simulink model "IEEE123_4subsystem"  (R2022b)
settings: Solver=ode4  StartTime=0.0  StopTime=inf  FixedStep=Ts  MaxStep=1e-4  RelTol=1e-3
PreLoadFcn:
  | Ts = 50e-6;
PostLoadFcn:
  | Ts = 50e-6;
InitFcn:
  | %%%%%%%%%%%%%%%%%%%%%%%%
  | % Simulation data for the IEEE 123 Node Test Feeder model
  | %%%%%%%%%%%%%%%%%%%%%%%
  | 
  | % miles/km
  | mi2km = 1.60934;
  | 
  | % feet to km
  | ft2km = 0.0003048;
  | 
  | % microsiemens to Farads
  | ms2F = 1/2/pi/60*1e-6;
  | 
  | %% Configuration 1 - series reactance - ohm/mile
  | 
  | R_1 = [0.4576 0.1560 0.1535;0.1560 0.4666 0.1580;0.1535 0.1580 0.4615];
  | X_1 = [1.0780 0.5017 0.3849;0.5017 1.0482 0.4236;0.3849 0.4236 1.0651];
  | 
  | % charging susceptance - microsiemens/mile
  | 
  | B_1 = [5.6765 -1.8319 -0.6982;-1.8319 5.9809 -1.1645;-0.6982 -1.1645 5.3971];
  | 
  | % convert for SPS
  | 
  | R_1 = R_1/mi2km;
  | 
  | Rs_1=(R_1(1,1)+R_1(2,2)+R_1(3,3))/3;
  | Rm_1=(R_1(1,2)+R_1(1,3)+R_1(2,3))/3;
  | R1_1=Rs_1-Rm_1;
  | R0_1=Rs_1+2*Rm_1;
  | 
  | L_1 = X_1/mi2km/2/pi/60;
  | 
  | Ls_1=(L_1(1,1)+L_1(2,2)+L_1(3,3))/3;
  | Lm_1=(L_1(1,2)+L_1(1,3)+L_1(2,3))/3;
  | L1_1=Ls_1-Lm_1;
  | L0_1=Ls_1+2*Lm_1;
  | 
  | C_1 = B_1/mi2km*ms2F;
  | 
  | Cs_1=(C_1(1,1)+C_1(2,2)+C_1(3,3))/3;
  | Cm_1=(C_1(1,2)+C_1(1,3)+C_1(2,3))/3;
  | C1_1=Cs_1-Cm_1;
  | C0_1=Cs_1+2*Cm_1;
  | 
  | 
  | %% Configuration 2 - series reactance - ohm/mile
  | 
  | R_2 = [0.4666 0.1580 0.1560;0.1580 0.4615 0.1535;0.1560 0.1535 0.4576];
  | X_2 = [1.0482 0.4236 0.5017;0.4236 1.0651 0.3849;0.5017 0.3849 1.0780];
  | 
  | % charging susceptance - microsiemens/mile
  | 
  | B_2 = [5.9809 -1.1645 -1.8319;-1.1645 5.3971 -0.6982;-1.8319 -0.6982 5.6765];
  | 
  | % convert for SPS
  | 
  | R_2 = R_2/mi2km;
  | 
  | Rs_2=(R_2(1,1)+R_2(2,2)+R_2(3,3))/3;
  | ... (+341 lines)
undefined symbols (not defined in the file): D1, Delta, find_system, I, Left, MOV_segment9, powergui, Right, type, V, X
libraries: spsGroundLib x242, spsThreePhaseVIMeasurementLib x134, spsSeriesRLCBranchLib x107, spsSeriesRLCLoadLib x83, spsPiSectionLineLib x61, spsThreePhasePISectionLineLib x60, spsVoltageMeasurementLib x52, spsDCVoltageSourceLib x36, ssn_lib x28, artemis x24, spsACCurrentSourceLib x18, spsOnDelayLib x18
(part 11 of 15)

== system IEEE123_4subsystem/SM_123p/Regulator 1 Three Phase Ganged SVR/Single Phase SVR_A/Voltage Regulator Control/Tap Changer Control ==
  "Up " : Inport
  "Down " : Inport  Port=2
  Constant : Constant  Value=-1
  Constant1 : Constant
  Determine tap position : Subsystem
  Edge Detector : Subsystem  DialogController=POWERSYS.PowerSysDialog  mask(Edge Detector){model=Rising, ic=0}
      mask prompts: model "Edge:"; ic "Input at t = -eps:"
      mask help:
      | This block compares its present input to its previous input.
      |
      | If the input  is a logic signal (TRUE (1) or FALSE (0), the output is a one-step boolean signal TRUE  when  the specified edge (Rising, Falling or Either)  is detected.
      |
      | This block can also be used to detect the slope polarity of a continuous signal. For example, if the specified edge is  "Rising", the output is TRUE as long as the slope of the input signal is positive.
      |
      | The input value at time preceding t=0 is specified by the parameter "Input at t=-eps"
      mask init:
      | if model~=3,
      | 	x1 = (model -1)*20;
      |     x2 = (model -1)*60;
      | 	X1=[5,20,20,35]+25; Y1=[20+x2,20+x2,80-x2,80-x2];
      | 	X2=[5,20,35]+25;    Y2=[40+x1,60-x1,40+x1];
      | 	X3=[];X4=[];Y3=[];Y4=[];
      | else
      | 	x1 = 20;
      | 	x2 = 60;
      | 	X1=[5,20,20,35]+8; Y1=[20,20,80,80];
      | 	X2=[5,20,35]+8;    Y2=[40,60,40];
      | 	X3=[5,20,20,35]+53; Y3=[20+x2,20+x2,80-x2,80-x2];
      | 	X4=[5,20,35]+53;    Y4=[40+x1,60-x1,40+x1];
      | end
      | power_initmask();
      mask Help: This block is part of a subset of blocks in the Extras library that does not have documentation associated with it, other than the block mask description.
      mask TypeOptions model: Rising | Falling | Either
      mask Display: plot(0,0,100,100, X1,Y1,X2,Y2,X3,Y3,X4,Y4);
  Logical Operator : Logic  Operator=OR  AllPortsSameDT=off
  Logical Operator1 : Logic  AllPortsSameDT=off
  Mechanical Delay : TransportDelay  DelayTime=MecDelay  InitialOutput=InitialPosition  BufferSize=5120
  Memory : Memory  InitialCondition=1  InheritSampleTime=on
  Relational Operator : RelationalOperator  Operator===  OutDataTypeStr=float('double')  InputSameDT=off
  Switch : Switch  Threshold=0.5  InputSameDT=off
  TapNo : Outport  VectorParamsAs1DForOutWhenUnconnected=off
  Ready : Outport  Port=2  VectorParamsAs1DForOutWhenUnconnected=off
  wires:
  Edge Detector/1(Out) -> Logical Operator1/2
  Logical Operator/1 -> Edge Detector/1(In)
  Memory/1 -> Ready/1, Logical Operator1/1
  Relational Operator/1 -> Memory/1
  Determine tap position/1(TapNo) -> Relational Operator/1, Mechanical Delay/1
  Switch/1 -> Determine tap position/1(NewTap)
  Constant1/1 -> Switch/3
  Constant/1 -> Switch/1
  "Down "/1 -> Switch/2, Logical Operator/2
  "Up "/1 -> Logical Operator/1
  Logical Operator1/1 -> Determine tap position/Trigger
  Mechanical Delay/1 -> Relational Operator/2, TapNo/1

== system IEEE123_4subsystem/SM_123p/Regulator 1 Three Phase Ganged SVR/Single Phase SVR_A/Voltage Regulator Control/Voltage regulator ==
  Vmes (pu) : Inport
  Ready : Inport  Port=2
  RegOn : Inport  Port=3
  Dead Zone : DeadZone  LowerValue=-DeadBand/2  UpperValue=+DeadBand/2
  Discrete Variable Time Delay : spsDiscreteVariableTimeDelayLib/Discrete Variable Time Delay  MaxDelay=3/60+Ts  InitialValue=1  Ts=Ts  DFT=on
      settings: LibrarySourceBlock=|
      | sps_lib/Control/Discrete Variable
      | Time Delay
  Logical Operator : Logic  AllPortsSameDT=off
  Logical Operator1 : Logic  AllPortsSameDT=off
  On Delay : spsOnDelayLib/On Delay  DelayType=On delay  delay=TimeDelay  ic=0  Ts=Ts
  On Delay1 : spsOnDelayLib/On Delay  DelayType=On delay  delay=TimeDelay  ic=0  Ts=Ts
  Relational Operator : RelationalOperator  Operator=>  InputSameDT=off
  Relational Operator1 : RelationalOperator  Operator=<  InputSameDT=off
  Sum : Sum  Inputs=|+-  SaturateOnIntegerOverflow=on
  Switch : Switch  Threshold=1.5  InputSameDT=off
  Vref : Constant  Value=Vref
  Vref1 : Constant  Value=0
  Vref2 : Constant  Value=0
  Vref3 : Constant  Value=0
  Vref4 : Constant  Value=3/60
  Up : Outport  VectorParamsAs1DForOutWhenUnconnected=off
  Down : Outport  Port=2  VectorParamsAs1DForOutWhenUnconnected=off
  wires:
  Vref4/1 -> Discrete Variable Time Delay/2
  Discrete Variable Time Delay/1 -> Logical Operator/2, Logical Operator1/1
  Vref3/1 -> Relational Operator1/2
  On Delay1/1 -> Down/1
  Logical Operator1/1 -> On Delay1/1
  Relational Operator1/1 -> Logical Operator1/2
  On Delay/1 -> Up/1
  Logical Operator/1 -> On Delay/1
  Ready/1 -> Discrete Variable Time Delay/1
  Relational Operator/1 -> Logical Operator/1
  Vref1/1 -> Relational Operator/2
  Dead Zone/1 -> Relational Operator/1, Relational Operator1/1
  Vmes (pu)/1 -> Sum/2
  Vref/1 -> Sum/1
  Sum/1 -> Switch/1
  Switch/1 -> Dead Zone/1
  RegOn/1 -> Switch/2
  Vref2/1 -> Switch/3

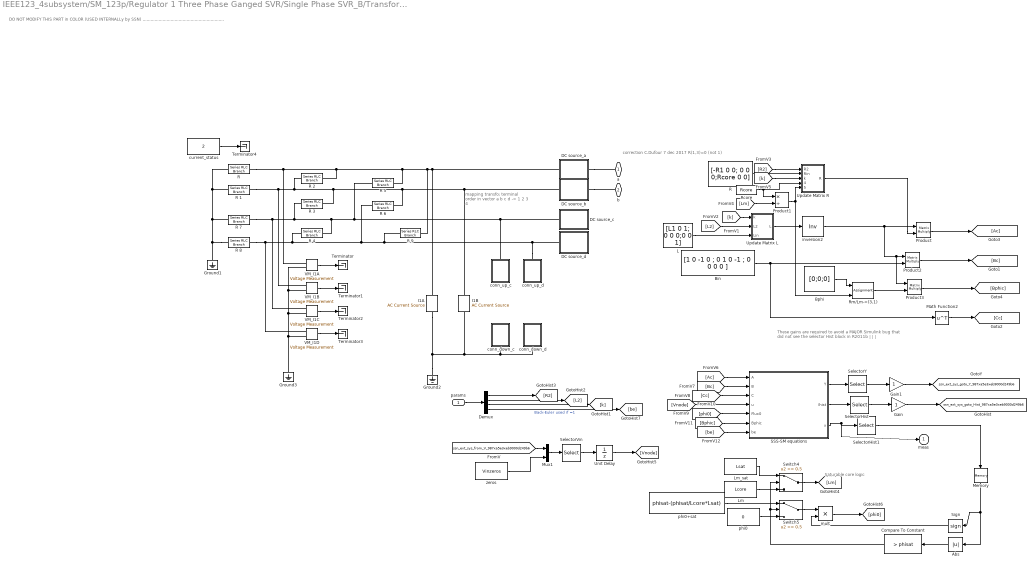
== system IEEE123_4subsystem/SM_123p/Regulator 1 Three Phase Ganged SVR/Single Phase SVR_B/Transformer with Taps/SSN OLTC xfo v2 ==
  note: correction C.Dufour 7 dec 2017 R(1,3)=0 (not 1)
  note: These gains are required to avoid a MAJOR Simulink bug
      | that did not see the selector Hist block in R2011b
      | |
      | |
      | |
  note: Saturable core logic
  note: DO NOT MODIFY THIS PART in COLOR (USED INTERNALLy by SSN) .............................................................
  note: mapping transfo:
      | terminal    order in vector
      | a b c d -> 1 2 3 4
  params : Inport
  Abs : Abs  SaturateOnIntegerOverflow=off
  Bin : Constant  Value="[1 0 -1  0 ; 0 1 0 -1 ; 0 0 0 0 ]"
  Bphi : Constant  Value=[0;0;0]  VectorParams1D=off
  Compare To Constant : simulink/Logic and Bit Operations/Compare To Constant  relop=>  const=phisat  OutDataTypeStr=uint8
  DC source_a : Subsystem  mask(SSN nodal point interface: DC-source){}
  DC source_b : Subsystem  mask(SSN nodal point interface: DC-source){}
  DC source_c : Subsystem  mask(SSN nodal point interface: DC-source){}
  DC source_d : Subsystem  mask(SSN nodal point interface: DC-source){}
  Demux : Demux
  Gain : Gain
  Gain1 : Gain
  Ground1 : spsGroundLib/Ground  LConnTagsString=a
  Ground2 : spsGroundLib/Ground  LConnTagsString=a
  Ground3 : spsGroundLib/Ground  LConnTagsString=a
  I1A : spsACCurrentSourceLib/AC Current Source  Amplitude=0  Phase=0  Frequency=1928.3746  SampleTime=0  Measurements=None
      settings: LibrarySourceBlock=sps_lib/Sources/AC Current Source
  I1B : spsACCurrentSourceLib/AC Current Source  Amplitude=0  Phase=0  Frequency=1928.3746  SampleTime=0  Measurements=None
      settings: LibrarySourceBlock=sps_lib/Sources/AC Current Source
  L : Constant  Value=[L1 0 1; 0 0 0;0 0 1]
  Lm : Constant  Value=Lcore
  Lm_sat : Constant  Value=Lsat
  Math Function2 : Math  Operator=transpose  SignedPower=on
  Memory : Memory
  Mux1 : Mux  Inputs=2
  Product : Product  Multiplication=Matrix(*)  RndMeth=Zero
  Product1 : Product  Inputs=*/  RndMeth=Zero
  Product2 : Product  Multiplication=Matrix(*)  RndMeth=Zero
  Product3 : Product  Multiplication=Matrix(*)  RndMeth=Zero
  R : Constant  Value=[-R1 0 0; 0 0 0;Rcore 0 0]
  R {,1..9} (10 alike) : spsSeriesRLCBranchLib/Series RLC Branch  LConnTagsString=__new0  RConnTagsString=__new0  BranchType=R  Resistance=1.23456789  Inductance=.5  SetiL0=off  InitialCurrent=0  Capacitance=1.0  Setx0=off  InitialVoltage=0  Measurements=None
  Rcore : Constant  Value=Rcore
  "Rm/Lm->(3,1) " : Assignment  NumberOfDimensions=2  IndexOptions=Index vector (dialog),Index vector (dialog)  Indices=3,1  OutputSizes=1,1
  SSS-SM equations : Subsystem
  SelectorHist : Selector  InputPortWidth=4  IndexOptions=Index vector (dialog)  Indices=hist_sel  OutputSizes=1
  SelectorHist1 : Selector  InputPortWidth=3  IndexOptions=Index vector (dialog)  Indices=3  OutputSizes=1
  SelectorVin : Selector  InputPortWidth=5  IndexOptions=Index vector (dialog)  Indices=vin_sel  OutputSizes=1
  SelectorY : Selector  NumberOfDimensions=2  InputPortWidth=4  IndexOptions=Index vector (dialog),Index vector (dialog)  Indices=hist_sel,hist_sel  OutputSizes=1,1
  Sign : Signum
  Switch4 : Switch  Threshold=0.5  SaturateOnIntegerOverflow=off  InputSameDT=off
  Switch5 : Switch  Threshold=0.5  SaturateOnIntegerOverflow=off  InputSameDT=off
  Terminator{,1..4} (5 alike) : Terminator
  Unit Delay : UnitDelay  SampleTime=Ts  HasFrameUpgradeWarning=on
  Update Matrix L : Subsystem
  Update Matrix R : Subsystem
  VM_I1A : spsVoltageMeasurementLib/Voltage Measurement  PhasorSimulation=off  OutputType=Complex  PSBequivalent=0
  VM_I1B : spsVoltageMeasurementLib/Voltage Measurement  PhasorSimulation=off  OutputType=Complex  PSBequivalent=0
  VM_I1C : spsVoltageMeasurementLib/Voltage Measurement  PhasorSimulation=off  OutputType=Complex  PSBequivalent=0
  VM_I1D : spsVoltageMeasurementLib/Voltage Measurement  PhasorSimulation=off  OutputType=Complex  PSBequivalent=0
  conn_down_c : Subsystem
  conn_down_d : Subsystem
  conn_up_c : Subsystem
  conn_up_d : Subsystem
  current_status : Constant  Value=2
  inversion2 : Product  Inputs=/  Multiplication=Matrix(*)  RndMeth=Zero
  mult : Product
  phi0 : Constant  Value=0
  phi0+sat : Constant  Value=phisat-(phisat/Lcore*Lsat)
  zeros : Constant  Value=Vinzeros
  a : PMIOPort  Side=Left
  b : PMIOPort  Port=2  Side=Right
  meas : Outport  InitialOutput=0  VectorParamsAs1DForOutWhenUnconnected=off
  tag scope: ssn_ext_sys_goto_Hist_987xa5e3xeb9000d249b6=global, ssn_ext_sys_goto_Y_987xa5e3xeb9000d249b6=global
  wires:
  Gain1/1 -> [ssn_ext_sys_goto_Y_987xa5e3xeb9000d249b6]
  Gain/1 -> [ssn_ext_sys_goto_Hist_987xa5e3xeb9000d249b6]
  Sign/1 -> mult/2
  mult/1 -> [phi0]
  Switch5/1 -> mult/1
  Unit Delay/1 -> [Vnode]
  params/1 -> Demux/1
  Demux/1 -> [R2]
  Demux/2 -> [L2]
  Demux/3 -> [k]
  Abs/1 -> Compare To Constant/1
  Lm_sat/1 -> Switch4/1
  Lm/1 -> Switch4/3
  Memory/1 -> Abs/1, Sign/1
  phi0/1 -> Switch5/3
  phi0+sat/1 -> Switch5/1
  Switch4/1 -> [Lm]
  Compare To Constant/1 -> Switch4/2, Switch5/2
  [ssn_ext_sys_from_V_987xa5e3xeb9000d249b6] -> Mux1/1
  zeros/1 -> Mux1/2
  SelectorVin/1 -> Unit Delay/1
  Mux1/1 -> SelectorVin/1
  current_status/1 -> Terminator4/1
  VM_I1D/1 -> Terminator3/1
  VM_I1C/1 -> Terminator2/1
  VM_I1B/1 -> Terminator1/1
  VM_I1A/1 -> Terminator/1
  L/1 -> Update Matrix L/3(Lin)
  [k] -> Update Matrix L/1(k)
  [L2] -> Update Matrix L/2(L2)
  Update Matrix L/1(L) -> inversion2/1
  R/1 -> Update Matrix R/2(Rin)
  [R2] -> Update Matrix R/1(R2)
  [k] -> Update Matrix R/3(k)
  Rcore/1 -> Update Matrix R/4(Rcore), Product1/1
  inversion2/1 -> Product2/1, Product3/1, Product/1
  [Lm] -> Product1/2
  Product1/1 -> Update Matrix R/5(Rcore/Lcore), "Rm/Lm->(3,1) "/2
  Bin/1 -> Math Function2/1, Product2/2
  Math Function2/1 -> [Cc]
  [Ac] -> SSS-SM equations/1(A)
  [Bc] -> SSS-SM equations/2(B)
  [Cc] -> SSS-SM equations/3(C)
  [Vnode] -> SSS-SM equations/4(u)
  [phi0] -> SSS-SM equations/5(Flux0)
  Bphi/1 -> "Rm/Lm->(3,1) "/1
  [Bphic] -> SSS-SM equations/6(Bphic)
  Product2/1 -> [Bc]
  "Rm/Lm->(3,1) "/1 -> Product3/2
  Update Matrix R/1(R) -> Product/2
  Product/1 -> [Ac]
  Product3/1 -> [Bphic]
  SSS-SM equations/3(x) -> SelectorHist1/1, meas/1
  SelectorHist1/1 -> Memory/1
  [be] -> SSS-SM equations/7(be)
  Demux/4 -> [be]  "Back-Euler used if =1"
  SSS-SM equations/2(Ihist) -> SelectorHist/1
  SSS-SM equations/1(Y) -> SelectorY/1
  SelectorY/1 -> Gain1/1
  SelectorHist/1 -> Gain/1
  connections:
  R 5/RConn1 -- VM_I1A/LConn1 -- "R "/RConn1 -- R 2/RConn1 -- I1A/RConn1 -- DC source_a/LConn1 -- R 9/RConn1
  R 3/RConn1 -- VM_I1B/LConn1 -- R 1/RConn1 -- R 2/LConn1 -- I1B/RConn1 -- DC source_b/LConn1 -- R 6/RConn1
  R 4/RConn1 -- VM_I1C/LConn1 -- R 7/RConn1 -- R 3/LConn1 -- conn_up_c/LConn1 -- DC source_c/LConn1 -- R 5/LConn1
  conn_up_d/LConn1 -- DC source_d/LConn1 -- R 9/LConn1 -- R 6/LConn1 -- VM_I1D/LConn1 -- R 8/RConn1 -- R 4/LConn1
  Ground3/LConn1 -- VM_I1C/LConn2 -- VM_I1A/LConn2 -- VM_I1B/LConn2 -- VM_I1D/LConn2
  DC source_b/RConn1 -- b/RConn1
  Ground2/LConn1 -- I1A/LConn1 -- I1B/LConn1 -- conn_down_c/RConn1 -- conn_down_d/RConn1
  DC source_a/RConn1 -- a/RConn1
  R 8/LConn1 -- Ground1/LConn1 -- R 7/LConn1 -- R 1/LConn1 -- "R "/LConn1

== system IEEE123_4subsystem/SM_123p/Regulator 1 Three Phase Ganged SVR/Single Phase SVR_B/Voltage Regulator Control/Tap Changer Control ==
  "Up " : Inport
  "Down " : Inport  Port=2
  Constant : Constant  Value=-1
  Constant1 : Constant
  Determine tap position : Subsystem
  Edge Detector : Subsystem  DialogController=POWERSYS.PowerSysDialog  mask(Edge Detector){model=Rising, ic=0}
      mask prompts: model "Edge:"; ic "Input at t = -eps:"
      mask help:
      | This block compares its present input to its previous input.
      |
      | If the input  is a logic signal (TRUE (1) or FALSE (0), the output is a one-step boolean signal TRUE  when  the specified edge (Rising, Falling or Either)  is detected.
      |
      | This block can also be used to detect the slope polarity of a continuous signal. For example, if the specified edge is  "Rising", the output is TRUE as long as the slope of the input signal is positive.
      |
      | The input value at time preceding t=0 is specified by the parameter "Input at t=-eps"
      mask init: same as IEEE123_4subsystem/SM_123p/Regulator 1 Three Phase Ganged SVR/Single Phase SVR_A/Voltage Regulator Control/Tap Changer Control/Edge Detector
      mask Help: This block is part of a subset of blocks in the Extras library that does not have documentation associated with it, other than the block mask description.
      mask TypeOptions model: Rising | Falling | Either
      mask Display: plot(0,0,100,100, X1,Y1,X2,Y2,X3,Y3,X4,Y4);
  Logical Operator : Logic  Operator=OR  AllPortsSameDT=off
  Logical Operator1 : Logic  AllPortsSameDT=off
  Mechanical Delay : TransportDelay  DelayTime=MecDelay  InitialOutput=InitialPosition  BufferSize=5120
  Memory : Memory  InitialCondition=1  InheritSampleTime=on
  Relational Operator : RelationalOperator  Operator===  OutDataTypeStr=float('double')  InputSameDT=off
  Switch : Switch  Threshold=0.5  InputSameDT=off
  TapNo : Outport  VectorParamsAs1DForOutWhenUnconnected=off
  Ready : Outport  Port=2  VectorParamsAs1DForOutWhenUnconnected=off
  wires:
  Edge Detector/1(Out) -> Logical Operator1/2
  Logical Operator/1 -> Edge Detector/1(In)
  Memory/1 -> Ready/1, Logical Operator1/1
  Relational Operator/1 -> Memory/1
  Determine tap position/1(TapNo) -> Relational Operator/1, Mechanical Delay/1
  Switch/1 -> Determine tap position/1(NewTap)
  Constant1/1 -> Switch/3
  Constant/1 -> Switch/1
  "Down "/1 -> Switch/2, Logical Operator/2
  "Up "/1 -> Logical Operator/1
  Logical Operator1/1 -> Determine tap position/Trigger
  Mechanical Delay/1 -> Relational Operator/2, TapNo/1

== system IEEE123_4subsystem/SM_123p/Regulator 1 Three Phase Ganged SVR/Single Phase SVR_B/Voltage Regulator Control/Voltage regulator ==
  Vmes (pu) : Inport
  Ready : Inport  Port=2
  RegOn : Inport  Port=3
  Dead Zone : DeadZone  LowerValue=-DeadBand/2  UpperValue=+DeadBand/2
  Discrete Variable Time Delay : spsDiscreteVariableTimeDelayLib/Discrete Variable Time Delay  MaxDelay=3/60+Ts  InitialValue=1  Ts=Ts  DFT=on
      settings: LibrarySourceBlock=|
      | sps_lib/Control/Discrete Variable
      | Time Delay
  Logical Operator : Logic  AllPortsSameDT=off
  Logical Operator1 : Logic  AllPortsSameDT=off
  On Delay : spsOnDelayLib/On Delay  DelayType=On delay  delay=TimeDelay  ic=0  Ts=Ts
  On Delay1 : spsOnDelayLib/On Delay  DelayType=On delay  delay=TimeDelay  ic=0  Ts=Ts
  Relational Operator : RelationalOperator  Operator=>  InputSameDT=off
  Relational Operator1 : RelationalOperator  Operator=<  InputSameDT=off
  Sum : Sum  Inputs=|+-  SaturateOnIntegerOverflow=on
  Switch : Switch  Threshold=1.5  InputSameDT=off
  Vref : Constant  Value=Vref
  Vref1 : Constant  Value=0
  Vref2 : Constant  Value=0
  Vref3 : Constant  Value=0
  Vref4 : Constant  Value=3/60
  Up : Outport  VectorParamsAs1DForOutWhenUnconnected=off
  Down : Outport  Port=2  VectorParamsAs1DForOutWhenUnconnected=off
  wires:
  Vref4/1 -> Discrete Variable Time Delay/2
  Discrete Variable Time Delay/1 -> Logical Operator/2, Logical Operator1/1
  Vref3/1 -> Relational Operator1/2
  On Delay1/1 -> Down/1
  Logical Operator1/1 -> On Delay1/1
  Relational Operator1/1 -> Logical Operator1/2
  On Delay/1 -> Up/1
  Logical Operator/1 -> On Delay/1
  Ready/1 -> Discrete Variable Time Delay/1
  Relational Operator/1 -> Logical Operator/1
  Vref1/1 -> Relational Operator/2
  Dead Zone/1 -> Relational Operator/1, Relational Operator1/1
  Vmes (pu)/1 -> Sum/2
  Vref/1 -> Sum/1
  Sum/1 -> Switch/1
  Switch/1 -> Dead Zone/1
  RegOn/1 -> Switch/2
  Vref2/1 -> Switch/3

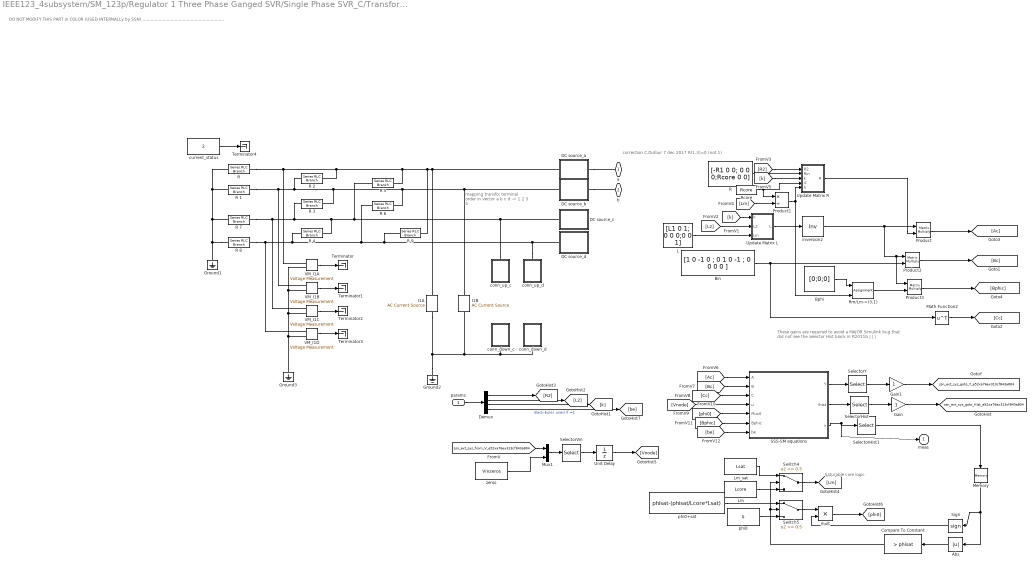
== system IEEE123_4subsystem/SM_123p/Regulator 1 Three Phase Ganged SVR/Single Phase SVR_C/Transformer with Taps/SSN OLTC xfo v2 ==
  note: correction C.Dufour 7 dec 2017 R(1,3)=0 (not 1)
  note: These gains are required to avoid a MAJOR Simulink bug
      | that did not see the selector Hist block in R2011b
      | |
      | |
      | |
  note: Saturable core logic
  note: DO NOT MODIFY THIS PART in COLOR (USED INTERNALLy by SSN) .............................................................
  note: mapping transfo:
      | terminal    order in vector
      | a b c d -> 1 2 3 4
  params : Inport
  Abs : Abs  SaturateOnIntegerOverflow=off
  Bin : Constant  Value="[1 0 -1  0 ; 0 1 0 -1 ; 0 0 0 0 ]"
  Bphi : Constant  Value=[0;0;0]  VectorParams1D=off
  Compare To Constant : simulink/Logic and Bit Operations/Compare To Constant  relop=>  const=phisat  OutDataTypeStr=uint8
  DC source_a : Subsystem  mask(SSN nodal point interface: DC-source){}
  DC source_b : Subsystem  mask(SSN nodal point interface: DC-source){}
  DC source_c : Subsystem  mask(SSN nodal point interface: DC-source){}
  DC source_d : Subsystem  mask(SSN nodal point interface: DC-source){}
  Demux : Demux
  Gain : Gain
  Gain1 : Gain
  Ground1 : spsGroundLib/Ground  LConnTagsString=a
  Ground2 : spsGroundLib/Ground  LConnTagsString=a
  Ground3 : spsGroundLib/Ground  LConnTagsString=a
  I1A : spsACCurrentSourceLib/AC Current Source  Amplitude=0  Phase=0  Frequency=1928.3746  SampleTime=0  Measurements=None
      settings: LibrarySourceBlock=sps_lib/Sources/AC Current Source
  I1B : spsACCurrentSourceLib/AC Current Source  Amplitude=0  Phase=0  Frequency=1928.3746  SampleTime=0  Measurements=None
      settings: LibrarySourceBlock=sps_lib/Sources/AC Current Source
  L : Constant  Value=[L1 0 1; 0 0 0;0 0 1]
  Lm : Constant  Value=Lcore
  Lm_sat : Constant  Value=Lsat
  Math Function2 : Math  Operator=transpose  SignedPower=on
  Memory : Memory
  Mux1 : Mux  Inputs=2
  Product : Product  Multiplication=Matrix(*)  RndMeth=Zero
  Product1 : Product  Inputs=*/  RndMeth=Zero
  Product2 : Product  Multiplication=Matrix(*)  RndMeth=Zero
  Product3 : Product  Multiplication=Matrix(*)  RndMeth=Zero
  R : Constant  Value=[-R1 0 0; 0 0 0;Rcore 0 0]
  R {,1..9} (10 alike) : spsSeriesRLCBranchLib/Series RLC Branch  LConnTagsString=__new0  RConnTagsString=__new0  BranchType=R  Resistance=1.23456789  Inductance=.5  SetiL0=off  InitialCurrent=0  Capacitance=1.0  Setx0=off  InitialVoltage=0  Measurements=None
  Rcore : Constant  Value=Rcore
  "Rm/Lm->(3,1) " : Assignment  NumberOfDimensions=2  IndexOptions=Index vector (dialog),Index vector (dialog)  Indices=3,1  OutputSizes=1,1
  SSS-SM equations : Subsystem
  SelectorHist : Selector  InputPortWidth=4  IndexOptions=Index vector (dialog)  Indices=hist_sel  OutputSizes=1
  SelectorHist1 : Selector  InputPortWidth=3  IndexOptions=Index vector (dialog)  Indices=3  OutputSizes=1
  SelectorVin : Selector  InputPortWidth=5  IndexOptions=Index vector (dialog)  Indices=vin_sel  OutputSizes=1
  SelectorY : Selector  NumberOfDimensions=2  InputPortWidth=4  IndexOptions=Index vector (dialog),Index vector (dialog)  Indices=hist_sel,hist_sel  OutputSizes=1,1
  Sign : Signum
  Switch4 : Switch  Threshold=0.5  SaturateOnIntegerOverflow=off  InputSameDT=off
  Switch5 : Switch  Threshold=0.5  SaturateOnIntegerOverflow=off  InputSameDT=off
  Terminator{,1..4} (5 alike) : Terminator
  Unit Delay : UnitDelay  SampleTime=Ts  HasFrameUpgradeWarning=on
  Update Matrix L : Subsystem
  Update Matrix R : Subsystem
  VM_I1A : spsVoltageMeasurementLib/Voltage Measurement  PhasorSimulation=off  OutputType=Complex  PSBequivalent=0
  VM_I1B : spsVoltageMeasurementLib/Voltage Measurement  PhasorSimulation=off  OutputType=Complex  PSBequivalent=0
  VM_I1C : spsVoltageMeasurementLib/Voltage Measurement  PhasorSimulation=off  OutputType=Complex  PSBequivalent=0
  VM_I1D : spsVoltageMeasurementLib/Voltage Measurement  PhasorSimulation=off  OutputType=Complex  PSBequivalent=0
  conn_down_c : Subsystem
  conn_down_d : Subsystem
  conn_up_c : Subsystem
  conn_up_d : Subsystem
  current_status : Constant  Value=2
  inversion2 : Product  Inputs=/  Multiplication=Matrix(*)  RndMeth=Zero
  mult : Product
  phi0 : Constant  Value=0
  phi0+sat : Constant  Value=phisat-(phisat/Lcore*Lsat)
  zeros : Constant  Value=Vinzeros
  a : PMIOPort  Side=Left
  b : PMIOPort  Port=2  Side=Right
  meas : Outport  InitialOutput=0  VectorParamsAs1DForOutWhenUnconnected=off
  tag scope: ssn_ext_sys_goto_Hist_e52xa76ex313cf843a804=global, ssn_ext_sys_goto_Y_e52xa76ex313cf843a804=global
  wires:
  Gain1/1 -> [ssn_ext_sys_goto_Y_e52xa76ex313cf843a804]
  Gain/1 -> [ssn_ext_sys_goto_Hist_e52xa76ex313cf843a804]
  Sign/1 -> mult/2
  mult/1 -> [phi0]
  Switch5/1 -> mult/1
  Unit Delay/1 -> [Vnode]
  params/1 -> Demux/1
  Demux/1 -> [R2]
  Demux/2 -> [L2]
  Demux/3 -> [k]
  Abs/1 -> Compare To Constant/1
  Lm_sat/1 -> Switch4/1
  Lm/1 -> Switch4/3
  Memory/1 -> Abs/1, Sign/1
  phi0/1 -> Switch5/3
  phi0+sat/1 -> Switch5/1
  Switch4/1 -> [Lm]
  Compare To Constant/1 -> Switch4/2, Switch5/2
  [ssn_ext_sys_from_V_e52xa76ex313cf843a804] -> Mux1/1
  zeros/1 -> Mux1/2
  SelectorVin/1 -> Unit Delay/1
  Mux1/1 -> SelectorVin/1
  current_status/1 -> Terminator4/1
  VM_I1D/1 -> Terminator3/1
  VM_I1C/1 -> Terminator2/1
  VM_I1B/1 -> Terminator1/1
  VM_I1A/1 -> Terminator/1
  L/1 -> Update Matrix L/3(Lin)
  [k] -> Update Matrix L/1(k)
  [L2] -> Update Matrix L/2(L2)
  Update Matrix L/1(L) -> inversion2/1
  R/1 -> Update Matrix R/2(Rin)
  [R2] -> Update Matrix R/1(R2)
  [k] -> Update Matrix R/3(k)
  Rcore/1 -> Update Matrix R/4(Rcore), Product1/1
  inversion2/1 -> Product2/1, Product3/1, Product/1
  [Lm] -> Product1/2
  Product1/1 -> Update Matrix R/5(Rcore/Lcore), "Rm/Lm->(3,1) "/2
  Bin/1 -> Math Function2/1, Product2/2
  Math Function2/1 -> [Cc]
  [Ac] -> SSS-SM equations/1(A)
  [Bc] -> SSS-SM equations/2(B)
  [Cc] -> SSS-SM equations/3(C)
  [Vnode] -> SSS-SM equations/4(u)
  [phi0] -> SSS-SM equations/5(Flux0)
  Bphi/1 -> "Rm/Lm->(3,1) "/1
  [Bphic] -> SSS-SM equations/6(Bphic)
  Product2/1 -> [Bc]
  "Rm/Lm->(3,1) "/1 -> Product3/2
  Update Matrix R/1(R) -> Product/2
  Product/1 -> [Ac]
  Product3/1 -> [Bphic]
  SSS-SM equations/3(x) -> SelectorHist1/1, meas/1
  SelectorHist1/1 -> Memory/1
  [be] -> SSS-SM equations/7(be)
  Demux/4 -> [be]  "Back-Euler used if =1"
  SSS-SM equations/2(Ihist) -> SelectorHist/1
  SSS-SM equations/1(Y) -> SelectorY/1
  SelectorY/1 -> Gain1/1
  SelectorHist/1 -> Gain/1
  connections:
  R 5/RConn1 -- VM_I1A/LConn1 -- "R "/RConn1 -- R 2/RConn1 -- I1A/RConn1 -- DC source_a/LConn1 -- R 9/RConn1
  R 3/RConn1 -- VM_I1B/LConn1 -- R 1/RConn1 -- R 2/LConn1 -- I1B/RConn1 -- DC source_b/LConn1 -- R 6/RConn1
  R 4/RConn1 -- VM_I1C/LConn1 -- R 7/RConn1 -- R 3/LConn1 -- conn_up_c/LConn1 -- DC source_c/LConn1 -- R 5/LConn1
  conn_up_d/LConn1 -- DC source_d/LConn1 -- R 9/LConn1 -- R 6/LConn1 -- VM_I1D/LConn1 -- R 8/RConn1 -- R 4/LConn1
  Ground3/LConn1 -- VM_I1C/LConn2 -- VM_I1A/LConn2 -- VM_I1B/LConn2 -- VM_I1D/LConn2
  DC source_b/RConn1 -- b/RConn1
  Ground2/LConn1 -- I1A/LConn1 -- I1B/LConn1 -- conn_down_c/RConn1 -- conn_down_d/RConn1
  DC source_a/RConn1 -- a/RConn1
  R 8/LConn1 -- Ground1/LConn1 -- R 7/LConn1 -- R 1/LConn1 -- "R "/LConn1

== system IEEE123_4subsystem/SM_123p/Regulator 1 Three Phase Ganged SVR/Single Phase SVR_C/Voltage Regulator Control/Tap Changer Control ==
  "Up " : Inport
  "Down " : Inport  Port=2
  Constant : Constant  Value=-1
  Constant1 : Constant
  Determine tap position : Subsystem
  Edge Detector : Subsystem  DialogController=POWERSYS.PowerSysDialog  mask(Edge Detector){model=Rising, ic=0}
      mask prompts: model "Edge:"; ic "Input at t = -eps:"
      mask help:
      | This block compares its present input to its previous input.
      |
      | If the input  is a logic signal (TRUE (1) or FALSE (0), the output is a one-step boolean signal TRUE  when  the specified edge (Rising, Falling or Either)  is detected.
      |
      | This block can also be used to detect the slope polarity of a continuous signal. For example, if the specified edge is  "Rising", the output is TRUE as long as the slope of the input signal is positive.
      |
      | The input value at time preceding t=0 is specified by the parameter "Input at t=-eps"
      mask init: same as IEEE123_4subsystem/SM_123p/Regulator 1 Three Phase Ganged SVR/Single Phase SVR_A/Voltage Regulator Control/Tap Changer Control/Edge Detector
      mask Help: This block is part of a subset of blocks in the Extras library that does not have documentation associated with it, other than the block mask description.
      mask TypeOptions model: Rising | Falling | Either
      mask Display: plot(0,0,100,100, X1,Y1,X2,Y2,X3,Y3,X4,Y4);
  Logical Operator : Logic  Operator=OR  AllPortsSameDT=off
  Logical Operator1 : Logic  AllPortsSameDT=off
  Mechanical Delay : TransportDelay  DelayTime=MecDelay  InitialOutput=InitialPosition  BufferSize=5120
  Memory : Memory  InitialCondition=1  InheritSampleTime=on
  Relational Operator : RelationalOperator  Operator===  OutDataTypeStr=float('double')  InputSameDT=off
  Switch : Switch  Threshold=0.5  InputSameDT=off
  TapNo : Outport  VectorParamsAs1DForOutWhenUnconnected=off
  Ready : Outport  Port=2  VectorParamsAs1DForOutWhenUnconnected=off
  wires:
  Edge Detector/1(Out) -> Logical Operator1/2
  Logical Operator/1 -> Edge Detector/1(In)
  Memory/1 -> Ready/1, Logical Operator1/1
  Relational Operator/1 -> Memory/1
  Determine tap position/1(TapNo) -> Relational Operator/1, Mechanical Delay/1
  Switch/1 -> Determine tap position/1(NewTap)
  Constant1/1 -> Switch/3
  Constant/1 -> Switch/1
  "Down "/1 -> Switch/2, Logical Operator/2
  "Up "/1 -> Logical Operator/1
  Logical Operator1/1 -> Determine tap position/Trigger
  Mechanical Delay/1 -> Relational Operator/2, TapNo/1

== system IEEE123_4subsystem/SM_123p/Regulator 1 Three Phase Ganged SVR/Single Phase SVR_C/Voltage Regulator Control/Voltage regulator ==
  Vmes (pu) : Inport
  Ready : Inport  Port=2
  RegOn : Inport  Port=3
  Dead Zone : DeadZone  LowerValue=-DeadBand/2  UpperValue=+DeadBand/2
  Discrete Variable Time Delay : spsDiscreteVariableTimeDelayLib/Discrete Variable Time Delay  MaxDelay=3/60+Ts  InitialValue=1  Ts=Ts  DFT=on
      settings: LibrarySourceBlock=|
      | sps_lib/Control/Discrete Variable
      | Time Delay
  Logical Operator : Logic  AllPortsSameDT=off
  Logical Operator1 : Logic  AllPortsSameDT=off
  On Delay : spsOnDelayLib/On Delay  DelayType=On delay  delay=TimeDelay  ic=0  Ts=Ts
  On Delay1 : spsOnDelayLib/On Delay  DelayType=On delay  delay=TimeDelay  ic=0  Ts=Ts
  Relational Operator : RelationalOperator  Operator=>  InputSameDT=off
  Relational Operator1 : RelationalOperator  Operator=<  InputSameDT=off
  Sum : Sum  Inputs=|+-  SaturateOnIntegerOverflow=on
  Switch : Switch  Threshold=1.5  InputSameDT=off
  Vref : Constant  Value=Vref
  Vref1 : Constant  Value=0
  Vref2 : Constant  Value=0
  Vref3 : Constant  Value=0
  Vref4 : Constant  Value=3/60
  Up : Outport  VectorParamsAs1DForOutWhenUnconnected=off
  Down : Outport  Port=2  VectorParamsAs1DForOutWhenUnconnected=off
  wires:
  Vref4/1 -> Discrete Variable Time Delay/2
  Discrete Variable Time Delay/1 -> Logical Operator/2, Logical Operator1/1
  Vref3/1 -> Relational Operator1/2
  On Delay1/1 -> Down/1
  Logical Operator1/1 -> On Delay1/1
  Relational Operator1/1 -> Logical Operator1/2
  On Delay/1 -> Up/1
  Logical Operator/1 -> On Delay/1
  Ready/1 -> Discrete Variable Time Delay/1
  Relational Operator/1 -> Logical Operator/1
  Vref1/1 -> Relational Operator/2
  Dead Zone/1 -> Relational Operator/1, Relational Operator1/1
  Vmes (pu)/1 -> Sum/2
  Vref/1 -> Sum/1
  Sum/1 -> Switch/1
  Switch/1 -> Dead Zone/1
  RegOn/1 -> Switch/2
  Vref2/1 -> Switch/3

== system IEEE123_4subsystem/SM_123p/Regulator 2/Single Phase SVR_A/Transformer with Taps/SSN OLTC xfo v2 ==
  note: correction C.Dufour 7 dec 2017 R(1,3)=0 (not 1)
  note: These gains are required to avoid a MAJOR Simulink bug
      | that did not see the selector Hist block in R2011b
      | |
      | |
      | |
  note: Saturable core logic
  note: DO NOT MODIFY THIS PART in COLOR (USED INTERNALLy by SSN) .............................................................
  note: mapping transfo:
      | terminal    order in vector
      | a b c d -> 1 2 3 4
  params : Inport
  Abs : Abs  SaturateOnIntegerOverflow=off
  Bin : Constant  Value="[1 0 -1  0 ; 0 1 0 -1 ; 0 0 0 0 ]"
  Bphi : Constant  Value=[0;0;0]  VectorParams1D=off
  Compare To Constant : simulink/Logic and Bit Operations/Compare To Constant  relop=>  const=phisat  OutDataTypeStr=uint8
  DC source_a : Subsystem  mask(SSN nodal point interface: DC-source){}
  DC source_b : Subsystem  mask(SSN nodal point interface: DC-source){}
  DC source_c : Subsystem  mask(SSN nodal point interface: DC-source){}
  DC source_d : Subsystem  mask(SSN nodal point interface: DC-source){}
  Demux : Demux
  Gain : Gain
  Gain1 : Gain
  Ground1 : spsGroundLib/Ground  LConnTagsString=a
  Ground2 : spsGroundLib/Ground  LConnTagsString=a
  Ground3 : spsGroundLib/Ground  LConnTagsString=a
  I1A : spsACCurrentSourceLib/AC Current Source  Amplitude=0  Phase=0  Frequency=1928.3746  SampleTime=0  Measurements=None
      settings: LibrarySourceBlock=sps_lib/Sources/AC Current Source
  I1B : spsACCurrentSourceLib/AC Current Source  Amplitude=0  Phase=0  Frequency=1928.3746  SampleTime=0  Measurements=None
      settings: LibrarySourceBlock=sps_lib/Sources/AC Current Source
  L : Constant  Value=[L1 0 1; 0 0 0;0 0 1]
  Lm : Constant  Value=Lcore
  Lm_sat : Constant  Value=Lsat
  Math Function2 : Math  Operator=transpose  SignedPower=on
  Memory : Memory
  Mux1 : Mux  Inputs=2
  Product : Product  Multiplication=Matrix(*)  RndMeth=Zero
  Product1 : Product  Inputs=*/  RndMeth=Zero
  Product2 : Product  Multiplication=Matrix(*)  RndMeth=Zero
  Product3 : Product  Multiplication=Matrix(*)  RndMeth=Zero
  R : Constant  Value=[-R1 0 0; 0 0 0;Rcore 0 0]
  R {,1..9} (10 alike) : spsSeriesRLCBranchLib/Series RLC Branch  LConnTagsString=__new0  RConnTagsString=__new0  BranchType=R  Resistance=1.23456789  Inductance=.5  SetiL0=off  InitialCurrent=0  Capacitance=1.0  Setx0=off  InitialVoltage=0  Measurements=None
  Rcore : Constant  Value=Rcore
  "Rm/Lm->(3,1) " : Assignment  NumberOfDimensions=2  IndexOptions=Index vector (dialog),Index vector (dialog)  Indices=3,1  OutputSizes=1,1
  SSS-SM equations : Subsystem
  SelectorHist : Selector  InputPortWidth=4  IndexOptions=Index vector (dialog)  Indices=hist_sel  OutputSizes=1
  SelectorHist1 : Selector  InputPortWidth=3  IndexOptions=Index vector (dialog)  Indices=3  OutputSizes=1
  SelectorVin : Selector  InputPortWidth=5  IndexOptions=Index vector (dialog)  Indices=vin_sel  OutputSizes=1
  SelectorY : Selector  NumberOfDimensions=2  InputPortWidth=4  IndexOptions=Index vector (dialog),Index vector (dialog)  Indices=hist_sel,hist_sel  OutputSizes=1,1
  Sign : Signum
  Switch4 : Switch  Threshold=0.5  SaturateOnIntegerOverflow=off  InputSameDT=off
  Switch5 : Switch  Threshold=0.5  SaturateOnIntegerOverflow=off  InputSameDT=off
  Terminator{,1..4} (5 alike) : Terminator
  Unit Delay : UnitDelay  SampleTime=Ts  HasFrameUpgradeWarning=on
  Update Matrix L : Subsystem
  Update Matrix R : Subsystem
  VM_I1A : spsVoltageMeasurementLib/Voltage Measurement  PhasorSimulation=off  OutputType=Complex  PSBequivalent=0
  VM_I1B : spsVoltageMeasurementLib/Voltage Measurement  PhasorSimulation=off  OutputType=Complex  PSBequivalent=0
  VM_I1C : spsVoltageMeasurementLib/Voltage Measurement  PhasorSimulation=off  OutputType=Complex  PSBequivalent=0
  VM_I1D : spsVoltageMeasurementLib/Voltage Measurement  PhasorSimulation=off  OutputType=Complex  PSBequivalent=0
  conn_down_c : Subsystem
  conn_down_d : Subsystem
  conn_up_c : Subsystem
  conn_up_d : Subsystem
  current_status : Constant  Value=2
  inversion2 : Product  Inputs=/  Multiplication=Matrix(*)  RndMeth=Zero
  mult : Product
  phi0 : Constant  Value=0
  phi0+sat : Constant  Value=phisat-(phisat/Lcore*Lsat)
  zeros : Constant  Value=Vinzeros
  a : PMIOPort  Side=Left
  b : PMIOPort  Port=2  Side=Right
  meas : Outport  InitialOutput=0  VectorParamsAs1DForOutWhenUnconnected=off
  tag scope: ssn_ext_sys_goto_Hist_89bxbdb6x1398f6ae2864=global, ssn_ext_sys_goto_Y_89bxbdb6x1398f6ae2864=global
  wires:
  Gain1/1 -> [ssn_ext_sys_goto_Y_89bxbdb6x1398f6ae2864]
  Gain/1 -> [ssn_ext_sys_goto_Hist_89bxbdb6x1398f6ae2864]
  Sign/1 -> mult/2
  mult/1 -> [phi0]
  Switch5/1 -> mult/1
  Unit Delay/1 -> [Vnode]
  params/1 -> Demux/1
  Demux/1 -> [R2]
  Demux/2 -> [L2]
  Demux/3 -> [k]
  Abs/1 -> Compare To Constant/1
  Lm_sat/1 -> Switch4/1
  Lm/1 -> Switch4/3
  Memory/1 -> Abs/1, Sign/1
  phi0/1 -> Switch5/3
  phi0+sat/1 -> Switch5/1
  Switch4/1 -> [Lm]
  Compare To Constant/1 -> Switch4/2, Switch5/2
  [ssn_ext_sys_from_V_89bxbdb6x1398f6ae2864] -> Mux1/1
  zeros/1 -> Mux1/2
  SelectorVin/1 -> Unit Delay/1
  Mux1/1 -> SelectorVin/1
  current_status/1 -> Terminator4/1
  VM_I1D/1 -> Terminator3/1
  VM_I1C/1 -> Terminator2/1
  VM_I1B/1 -> Terminator1/1
  VM_I1A/1 -> Terminator/1
  L/1 -> Update Matrix L/3(Lin)
  [k] -> Update Matrix L/1(k)
  [L2] -> Update Matrix L/2(L2)
  Update Matrix L/1(L) -> inversion2/1
  R/1 -> Update Matrix R/2(Rin)
  [R2] -> Update Matrix R/1(R2)
  [k] -> Update Matrix R/3(k)
  Rcore/1 -> Update Matrix R/4(Rcore), Product1/1
  inversion2/1 -> Product2/1, Product3/1, Product/1
  [Lm] -> Product1/2
  Product1/1 -> Update Matrix R/5(Rcore/Lcore), "Rm/Lm->(3,1) "/2
  Bin/1 -> Math Function2/1, Product2/2
  Math Function2/1 -> [Cc]
  [Ac] -> SSS-SM equations/1(A)
  [Bc] -> SSS-SM equations/2(B)
  [Cc] -> SSS-SM equations/3(C)
  [Vnode] -> SSS-SM equations/4(u)
  [phi0] -> SSS-SM equations/5(Flux0)
  Bphi/1 -> "Rm/Lm->(3,1) "/1
  [Bphic] -> SSS-SM equations/6(Bphic)
  Product2/1 -> [Bc]
  "Rm/Lm->(3,1) "/1 -> Product3/2
  Update Matrix R/1(R) -> Product/2
  Product/1 -> [Ac]
  Product3/1 -> [Bphic]
  SSS-SM equations/3(x) -> SelectorHist1/1, meas/1
  SelectorHist1/1 -> Memory/1
  [be] -> SSS-SM equations/7(be)
  Demux/4 -> [be]  "Back-Euler used if =1"
  SSS-SM equations/2(Ihist) -> SelectorHist/1
  SSS-SM equations/1(Y) -> SelectorY/1
  SelectorY/1 -> Gain1/1
  SelectorHist/1 -> Gain/1
  connections:
  R 5/RConn1 -- VM_I1A/LConn1 -- "R "/RConn1 -- R 2/RConn1 -- I1A/RConn1 -- DC source_a/LConn1 -- R 9/RConn1
  R 3/RConn1 -- VM_I1B/LConn1 -- R 1/RConn1 -- R 2/LConn1 -- I1B/RConn1 -- DC source_b/LConn1 -- R 6/RConn1
  R 4/RConn1 -- VM_I1C/LConn1 -- R 7/RConn1 -- R 3/LConn1 -- conn_up_c/LConn1 -- DC source_c/LConn1 -- R 5/LConn1
  conn_up_d/LConn1 -- DC source_d/LConn1 -- R 9/LConn1 -- R 6/LConn1 -- VM_I1D/LConn1 -- R 8/RConn1 -- R 4/LConn1
  Ground3/LConn1 -- VM_I1C/LConn2 -- VM_I1A/LConn2 -- VM_I1B/LConn2 -- VM_I1D/LConn2
  DC source_b/RConn1 -- b/RConn1
  Ground2/LConn1 -- I1A/LConn1 -- I1B/LConn1 -- conn_down_c/RConn1 -- conn_down_d/RConn1
  DC source_a/RConn1 -- a/RConn1
  R 8/LConn1 -- Ground1/LConn1 -- R 7/LConn1 -- R 1/LConn1 -- "R "/LConn1

== system IEEE123_4subsystem/SM_123p/Regulator 2/Single Phase SVR_A/Voltage Regulator Control/Tap Changer Control ==
  "Up " : Inport
  "Down " : Inport  Port=2
  Constant : Constant  Value=-1
  Constant1 : Constant
  Determine tap position : Subsystem
  Edge Detector : Subsystem  DialogController=POWERSYS.PowerSysDialog  mask(Edge Detector){model=Rising, ic=0}
      mask prompts: model "Edge:"; ic "Input at t = -eps:"
      mask help:
      | This block compares its present input to its previous input.
      |
      | If the input  is a logic signal (TRUE (1) or FALSE (0), the output is a one-step boolean signal TRUE  when  the specified edge (Rising, Falling or Either)  is detected.
      |
      | This block can also be used to detect the slope polarity of a continuous signal. For example, if the specified edge is  "Rising", the output is TRUE as long as the slope of the input signal is positive.
      |
      | The input value at time preceding t=0 is specified by the parameter "Input at t=-eps"
      mask init: same as IEEE123_4subsystem/SM_123p/Regulator 1 Three Phase Ganged SVR/Single Phase SVR_A/Voltage Regulator Control/Tap Changer Control/Edge Detector
      mask Help: This block is part of a subset of blocks in the Extras library that does not have documentation associated with it, other than the block mask description.
      mask TypeOptions model: Rising | Falling | Either
      mask Display: plot(0,0,100,100, X1,Y1,X2,Y2,X3,Y3,X4,Y4);
  Logical Operator : Logic  Operator=OR  AllPortsSameDT=off
  Logical Operator1 : Logic  AllPortsSameDT=off
  Mechanical Delay : TransportDelay  DelayTime=MecDelay  InitialOutput=InitialPosition  BufferSize=5120
  Memory : Memory  InitialCondition=1  InheritSampleTime=on
  Relational Operator : RelationalOperator  Operator===  OutDataTypeStr=float('double')  InputSameDT=off
  Switch : Switch  Threshold=0.5  InputSameDT=off
  TapNo : Outport  VectorParamsAs1DForOutWhenUnconnected=off
  Ready : Outport  Port=2  VectorParamsAs1DForOutWhenUnconnected=off
  wires:
  Edge Detector/1(Out) -> Logical Operator1/2
  Logical Operator/1 -> Edge Detector/1(In)
  Memory/1 -> Ready/1, Logical Operator1/1
  Relational Operator/1 -> Memory/1
  Determine tap position/1(TapNo) -> Relational Operator/1, Mechanical Delay/1
  Switch/1 -> Determine tap position/1(NewTap)
  Constant1/1 -> Switch/3
  Constant/1 -> Switch/1
  "Down "/1 -> Switch/2, Logical Operator/2
  "Up "/1 -> Logical Operator/1
  Logical Operator1/1 -> Determine tap position/Trigger
  Mechanical Delay/1 -> Relational Operator/2, TapNo/1

== system IEEE123_4subsystem/SM_123p/Regulator 2/Single Phase SVR_A/Voltage Regulator Control/Voltage regulator ==
  Vmes (pu) : Inport
  Ready : Inport  Port=2
  RegOn : Inport  Port=3
  Dead Zone : DeadZone  LowerValue=-DeadBand/2  UpperValue=+DeadBand/2
  Discrete Variable Time Delay : spsDiscreteVariableTimeDelayLib/Discrete Variable Time Delay  MaxDelay=3/60+Ts  InitialValue=1  Ts=Ts  DFT=on
      settings: LibrarySourceBlock=|
      | sps_lib/Control/Discrete Variable
      | Time Delay
  Logical Operator : Logic  AllPortsSameDT=off
  Logical Operator1 : Logic  AllPortsSameDT=off
  On Delay : spsOnDelayLib/On Delay  DelayType=On delay  delay=TimeDelay  ic=0  Ts=Ts
  On Delay1 : spsOnDelayLib/On Delay  DelayType=On delay  delay=TimeDelay  ic=0  Ts=Ts
  Relational Operator : RelationalOperator  Operator=>  InputSameDT=off
  Relational Operator1 : RelationalOperator  Operator=<  InputSameDT=off
  Sum : Sum  Inputs=|+-  SaturateOnIntegerOverflow=on
  Switch : Switch  Threshold=1.5  InputSameDT=off
  Vref : Constant  Value=Vref
  Vref1 : Constant  Value=0
  Vref2 : Constant  Value=0
  Vref3 : Constant  Value=0
  Vref4 : Constant  Value=3/60
  Up : Outport  VectorParamsAs1DForOutWhenUnconnected=off
  Down : Outport  Port=2  VectorParamsAs1DForOutWhenUnconnected=off
  wires:
  Vref4/1 -> Discrete Variable Time Delay/2
  Discrete Variable Time Delay/1 -> Logical Operator/2, Logical Operator1/1
  Vref3/1 -> Relational Operator1/2
  On Delay1/1 -> Down/1
  Logical Operator1/1 -> On Delay1/1
  Relational Operator1/1 -> Logical Operator1/2
  On Delay/1 -> Up/1
  Logical Operator/1 -> On Delay/1
  Ready/1 -> Discrete Variable Time Delay/1
  Relational Operator/1 -> Logical Operator/1
  Vref1/1 -> Relational Operator/2
  Dead Zone/1 -> Relational Operator/1, Relational Operator1/1
  Vmes (pu)/1 -> Sum/2
  Vref/1 -> Sum/1
  Sum/1 -> Switch/1
  Switch/1 -> Dead Zone/1
  RegOn/1 -> Switch/2
  Vref2/1 -> Switch/3

== system IEEE123_4subsystem/SS_123p1/Regulator 4/Single Phase SVR_A/Transformer with Taps/SSN OLTC xfo v2 ==
  note: correction C.Dufour 7 dec 2017 R(1,3)=0 (not 1)
  note: These gains are required to avoid a MAJOR Simulink bug
      | that did not see the selector Hist block in R2011b
      | |
      | |
      | |
  note: Saturable core logic
  note: DO NOT MODIFY THIS PART in COLOR (USED INTERNALLy by SSN) .............................................................
  note: mapping transfo:
      | terminal    order in vector
      | a b c d -> 1 2 3 4
  params : Inport
  Abs : Abs  SaturateOnIntegerOverflow=off
  Bin : Constant  Value="[1 0 -1  0 ; 0 1 0 -1 ; 0 0 0 0 ]"
  Bphi : Constant  Value=[0;0;0]  VectorParams1D=off
  Compare To Constant : simulink/Logic and Bit Operations/Compare To Constant  relop=>  const=phisat  OutDataTypeStr=uint8
  DC source_a : Subsystem  mask(SSN nodal point interface: DC-source){}
  DC source_b : Subsystem  mask(SSN nodal point interface: DC-source){}
  DC source_c : Subsystem  mask(SSN nodal point interface: DC-source){}
  DC source_d : Subsystem  mask(SSN nodal point interface: DC-source){}
  Demux : Demux
  Gain : Gain
  Gain1 : Gain
  Ground1 : spsGroundLib/Ground  LConnTagsString=a
  Ground2 : spsGroundLib/Ground  LConnTagsString=a
  Ground3 : spsGroundLib/Ground  LConnTagsString=a
  I1A : spsACCurrentSourceLib/AC Current Source  Amplitude=0  Phase=0  Frequency=1928.3746  SampleTime=0  Measurements=None
      settings: LibrarySourceBlock=sps_lib/Sources/AC Current Source
  I1B : spsACCurrentSourceLib/AC Current Source  Amplitude=0  Phase=0  Frequency=1928.3746  SampleTime=0  Measurements=None
      settings: LibrarySourceBlock=sps_lib/Sources/AC Current Source
  L : Constant  Value=[L1 0 1; 0 0 0;0 0 1]
  Lm : Constant  Value=Lcore
  Lm_sat : Constant  Value=Lsat
  Math Function2 : Math  Operator=transpose  SignedPower=on
  Memory : Memory
  Mux1 : Mux  Inputs=2
  Product : Product  Multiplication=Matrix(*)  RndMeth=Zero
  Product1 : Product  Inputs=*/  RndMeth=Zero
  Product2 : Product  Multiplication=Matrix(*)  RndMeth=Zero
  Product3 : Product  Multiplication=Matrix(*)  RndMeth=Zero
  R : Constant  Value=[-R1 0 0; 0 0 0;Rcore 0 0]
  R {,1..9} (10 alike) : spsSeriesRLCBranchLib/Series RLC Branch  LConnTagsString=__new0  RConnTagsString=__new0  BranchType=R  Resistance=1.23456789  Inductance=.5  SetiL0=off  InitialCurrent=0  Capacitance=1.0  Setx0=off  InitialVoltage=0  Measurements=None
  Rcore : Constant  Value=Rcore
  "Rm/Lm->(3,1) " : Assignment  NumberOfDimensions=2  IndexOptions=Index vector (dialog),Index vector (dialog)  Indices=3,1  OutputSizes=1,1
  SSS-SM equations : Subsystem
  SelectorHist : Selector  InputPortWidth=4  IndexOptions=Index vector (dialog)  Indices=hist_sel  OutputSizes=1
  SelectorHist1 : Selector  InputPortWidth=3  IndexOptions=Index vector (dialog)  Indices=3  OutputSizes=1
  SelectorVin : Selector  InputPortWidth=5  IndexOptions=Index vector (dialog)  Indices=vin_sel  OutputSizes=1
  SelectorY : Selector  NumberOfDimensions=2  InputPortWidth=4  IndexOptions=Index vector (dialog),Index vector (dialog)  Indices=hist_sel,hist_sel  OutputSizes=1,1
  Sign : Signum
  Switch4 : Switch  Threshold=0.5  SaturateOnIntegerOverflow=off  InputSameDT=off
  Switch5 : Switch  Threshold=0.5  SaturateOnIntegerOverflow=off  InputSameDT=off
  Terminator{,1..4} (5 alike) : Terminator
  Unit Delay : UnitDelay  SampleTime=Ts  HasFrameUpgradeWarning=on
  Update Matrix L : Subsystem
  Update Matrix R : Subsystem
  VM_I1A : spsVoltageMeasurementLib/Voltage Measurement  PhasorSimulation=off  OutputType=Complex  PSBequivalent=0
  VM_I1B : spsVoltageMeasurementLib/Voltage Measurement  PhasorSimulation=off  OutputType=Complex  PSBequivalent=0
  VM_I1C : spsVoltageMeasurementLib/Voltage Measurement  PhasorSimulation=off  OutputType=Complex  PSBequivalent=0
  VM_I1D : spsVoltageMeasurementLib/Voltage Measurement  PhasorSimulation=off  OutputType=Complex  PSBequivalent=0
  conn_down_c : Subsystem
  conn_down_d : Subsystem
  conn_up_c : Subsystem
  conn_up_d : Subsystem
  current_status : Constant  Value=2
  inversion2 : Product  Inputs=/  Multiplication=Matrix(*)  RndMeth=Zero
  mult : Product
  phi0 : Constant  Value=0
  phi0+sat : Constant  Value=phisat-(phisat/Lcore*Lsat)
  zeros : Constant  Value=Vinzeros
  a : PMIOPort  Side=Left
  b : PMIOPort  Port=2  Side=Right
  meas : Outport  InitialOutput=0  VectorParamsAs1DForOutWhenUnconnected=off
  tag scope: ssn_ext_sys_goto_Hist_0bexa56ax8042611b062e=global, ssn_ext_sys_goto_Y_0bexa56ax8042611b062e=global
  wires:
  Gain1/1 -> [ssn_ext_sys_goto_Y_0bexa56ax8042611b062e]
  Gain/1 -> [ssn_ext_sys_goto_Hist_0bexa56ax8042611b062e]
  Sign/1 -> mult/2
  mult/1 -> [phi0]
  Switch5/1 -> mult/1
  Unit Delay/1 -> [Vnode]
  params/1 -> Demux/1
  Demux/1 -> [R2]
  Demux/2 -> [L2]
  Demux/3 -> [k]
  Abs/1 -> Compare To Constant/1
  Lm_sat/1 -> Switch4/1
  Lm/1 -> Switch4/3
  Memory/1 -> Abs/1, Sign/1
  phi0/1 -> Switch5/3
  phi0+sat/1 -> Switch5/1
  Switch4/1 -> [Lm]
  Compare To Constant/1 -> Switch4/2, Switch5/2
  [ssn_ext_sys_from_V_0bexa56ax8042611b062e] -> Mux1/1
  zeros/1 -> Mux1/2
  SelectorVin/1 -> Unit Delay/1
  Mux1/1 -> SelectorVin/1
  current_status/1 -> Terminator4/1
  VM_I1D/1 -> Terminator3/1
  VM_I1C/1 -> Terminator2/1
  VM_I1B/1 -> Terminator1/1
  VM_I1A/1 -> Terminator/1
  L/1 -> Update Matrix L/3(Lin)
  [k] -> Update Matrix L/1(k)
  [L2] -> Update Matrix L/2(L2)
  Update Matrix L/1(L) -> inversion2/1
  R/1 -> Update Matrix R/2(Rin)
  [R2] -> Update Matrix R/1(R2)
  [k] -> Update Matrix R/3(k)
  Rcore/1 -> Update Matrix R/4(Rcore), Product1/1
  inversion2/1 -> Product2/1, Product3/1, Product/1
  [Lm] -> Product1/2
  Product1/1 -> Update Matrix R/5(Rcore/Lcore), "Rm/Lm->(3,1) "/2
  Bin/1 -> Math Function2/1, Product2/2
  Math Function2/1 -> [Cc]
  [Ac] -> SSS-SM equations/1(A)
  [Bc] -> SSS-SM equations/2(B)
  [Cc] -> SSS-SM equations/3(C)
  [Vnode] -> SSS-SM equations/4(u)
  [phi0] -> SSS-SM equations/5(Flux0)
  Bphi/1 -> "Rm/Lm->(3,1) "/1
  [Bphic] -> SSS-SM equations/6(Bphic)
  Product2/1 -> [Bc]
  "Rm/Lm->(3,1) "/1 -> Product3/2
  Update Matrix R/1(R) -> Product/2
  Product/1 -> [Ac]
  Product3/1 -> [Bphic]
  SSS-SM equations/3(x) -> SelectorHist1/1, meas/1
  SelectorHist1/1 -> Memory/1
  [be] -> SSS-SM equations/7(be)
  Demux/4 -> [be]  "Back-Euler used if =1"
  SSS-SM equations/2(Ihist) -> SelectorHist/1
  SSS-SM equations/1(Y) -> SelectorY/1
  SelectorY/1 -> Gain1/1
  SelectorHist/1 -> Gain/1
  connections:
  R 5/RConn1 -- VM_I1A/LConn1 -- "R "/RConn1 -- R 2/RConn1 -- I1A/RConn1 -- DC source_a/LConn1 -- R 9/RConn1
  R 3/RConn1 -- VM_I1B/LConn1 -- R 1/RConn1 -- R 2/LConn1 -- I1B/RConn1 -- DC source_b/LConn1 -- R 6/RConn1
  R 4/RConn1 -- VM_I1C/LConn1 -- R 7/RConn1 -- R 3/LConn1 -- conn_up_c/LConn1 -- DC source_c/LConn1 -- R 5/LConn1
  conn_up_d/LConn1 -- DC source_d/LConn1 -- R 9/LConn1 -- R 6/LConn1 -- VM_I1D/LConn1 -- R 8/RConn1 -- R 4/LConn1
  Ground3/LConn1 -- VM_I1C/LConn2 -- VM_I1A/LConn2 -- VM_I1B/LConn2 -- VM_I1D/LConn2
  DC source_b/RConn1 -- b/RConn1
  Ground2/LConn1 -- I1A/LConn1 -- I1B/LConn1 -- conn_down_c/RConn1 -- conn_down_d/RConn1
  DC source_a/RConn1 -- a/RConn1
  R 8/LConn1 -- Ground1/LConn1 -- R 7/LConn1 -- R 1/LConn1 -- "R "/LConn1
